simulink model "CurrentTestSimulation"  (R2022a)
settings: Solver=VariableStepAuto  StartTime=0.0  StopTime=10.0  RelTol=1e-3
values from neighbouring files (symbols this model uses):
  module = struct(     'M_inv', M_inv,     'J_w', J_w,     'Kt', Kt,     'Kv', Kv,     'Res', Res,     'sysc', sysc,     'sysd', sysd,     'lqr_K', lqr_K,     'Kff', Kff,     'D_w', D_w,     'Ts', Ts,     'Vmax', Vmax,     'Imax', Imax )    [GetDiffSwerveModule.m]
settings Model: Creator=woz4t  LastModifiedBy=woz4t

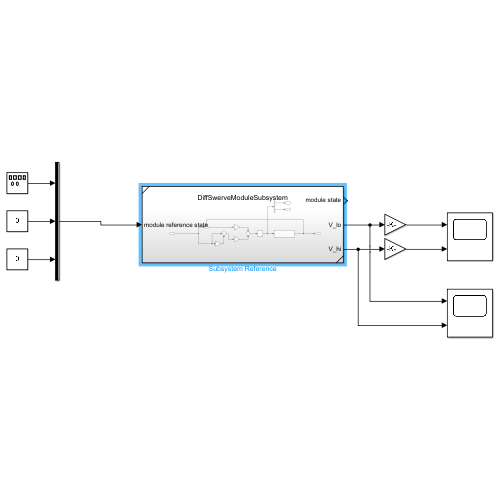
[thumbnail: Simulink's stored preview of the top-level diagram]
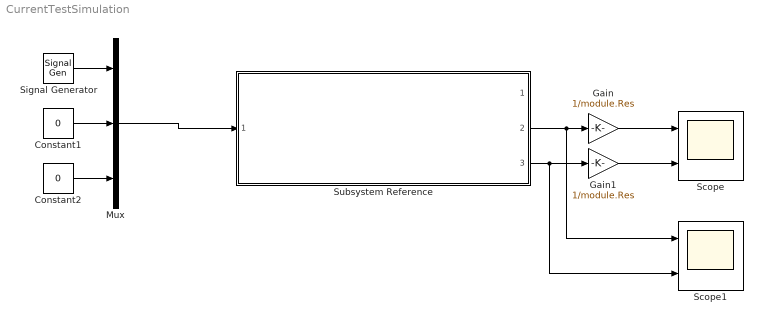
== system CurrentTestSimulation ==
  Constant1 : Constant  Value=0
  Constant2 : Constant  Value=0
  Gain : Gain  Gain=1/module.Res
  Gain1 : Gain  Gain=1/module.Res
  Mux : Mux  Inputs=3
  Scope : Scope  NumInputPorts=2
  Scope1 : Scope  NumInputPorts=2
  Signal Generator : SignalGenerator  WaveForm=square  Amplitude=5  Units=rad/sec
  Subsystem Reference : Subsystem  ReferencedSubsystem=DiffSwerveModuleSubsystem
  wires:
  Mux/1 -> Subsystem Reference/1
  Signal Generator/1 -> Mux/1
  Constant1/1 -> Mux/2
  Constant2/1 -> Mux/3
  Subsystem Reference/2 -> Gain/1, Scope1/1
  Subsystem Reference/3 -> Scope1/2, Gain1/1
  Gain/1 -> Scope/1
  Gain1/1 -> Scope/2
